simulink model "RABBIT_sfunction_test"  (R2015a)
settings: Solver=FixedStepDiscrete  StartTime=t_start  StopTime=t_end  FixedStep=dt  RelTol=1e-3
undefined symbols (not defined in the file or in its folder): dt
libraries: RABBIT_lib x2
settings Model: Creator=ffelici  LastModifiedBy=ffelici
settings OptimizationCC: OptimizeModelRefInitCode=on  LifeSpan=1
settings HardwareCC: TargetBitPerLong=64  TargetBitPerPointer=64  TargetLongLongMode=on  TargetIntDivRoundTo=Zero  TargetEndianess=LittleEndian  TargetWordSize=64  TargetHWDeviceType=MATLAB Host  ProdEqTarget=off
settings RTWCC: SystemTargetFile=ert_shrlib.tlc  TemplateMakefile=ert_unix_rabbit.tmf  Description=Embedded Coder (host-based shared library target)  RetainRTWFile=on  BuildConfiguration=Specify  RTWCompilerOptimization=Custom
settings CodeAppCC: IgnoreCustomStorageClasses=off
settings STFCustomTargetCC: GenerateSampleERTMain=off  ParMdlRefBuildCompliant=on  CompOptLevelCompliant=on  CombineOutputUpdateFcns=on  SupportContinuousTime=off  SupportNonInlinedSFcns=on  SupportVariableSizeSignals=off  ModelStepFunctionPrototypeControlCompliant=on  SystemTargetFile=ert_shrlib.tlc
settings ERTTargetCC: GenerateSampleERTMain=off  ParMdlRefBuildCompliant=on  CompOptLevelCompliant=on  SupportContinuousTime=off  SupportNonInlinedSFcns=on  SupportVariableSizeSignals=off  ModelStepFunctionPrototypeControlCompliant=on  ERTCustomFileTemplate=example_file_process.tlc

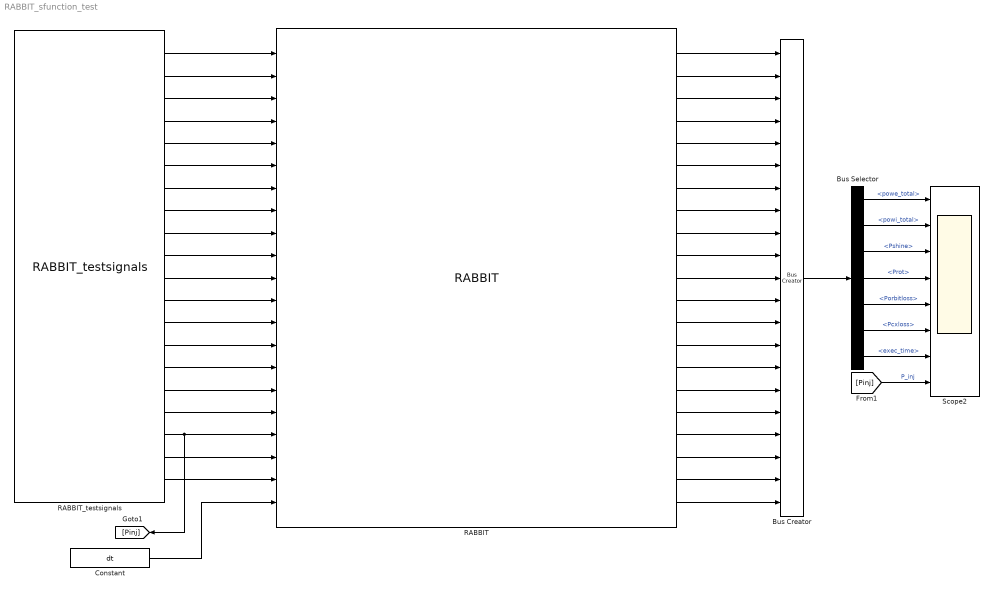
== system RABBIT_sfunction_test ==
  Bus Creator : BusCreator  Inputs=21
  Bus Selector : BusSelector  OutputSignals=powe_total,powi_total,Pshine,Prot,Porbitloss,Pcxloss,exec_time
  Constant : Constant  Value=dt
  RABBIT : RABBIT_lib/RABBIT  RABBITparams=RABBITparams
  RABBIT_testsignals : RABBIT_lib/RABBIT_testsignals  RABBITsignals=RABBITsignals  dt=dt
  Scope2 : Scope  NumInputPorts=8
      settings: YMin=0~0~600000~350000~-1~-1.25e-10~-1~-5  YMax=100000~250000~950000~550000~1~5e-11~1~5
  wires:
  Bus Selector/1 -> Scope2/1  "<powe_total>"
  Bus Selector/2 -> Scope2/2  "<powi_total>"
  Bus Selector/3 -> Scope2/3  "<Pshine>"
  Bus Selector/4 -> Scope2/4  "<Prot>"
  Bus Selector/5 -> Scope2/5  "<Porbitloss>"
  Bus Selector/6 -> Scope2/6  "<Pcxloss>"
  Bus Selector/7 -> Scope2/7  "<exec_time>"
  [Pinj] -> Scope2/8  "P_inj"
  Bus Creator/1 -> Bus Selector/1
  Constant/1 -> RABBIT/21
  RABBIT_testsignals/20 -> RABBIT/20
  RABBIT_testsignals/19 -> RABBIT/19
  RABBIT_testsignals/17 -> RABBIT/17
  RABBIT_testsignals/18 -> RABBIT/18, [Pinj]
  RABBIT_testsignals/16 -> RABBIT/16
  RABBIT_testsignals/15 -> RABBIT/15
  RABBIT_testsignals/14 -> RABBIT/14
  RABBIT_testsignals/13 -> RABBIT/13
  RABBIT_testsignals/12 -> RABBIT/12
  RABBIT_testsignals/11 -> RABBIT/11
  RABBIT_testsignals/10 -> RABBIT/10
  RABBIT_testsignals/9 -> RABBIT/9
  RABBIT_testsignals/8 -> RABBIT/8
  RABBIT_testsignals/7 -> RABBIT/7
  RABBIT_testsignals/6 -> RABBIT/6
  RABBIT_testsignals/4 -> RABBIT/4
  RABBIT_testsignals/5 -> RABBIT/5
  RABBIT_testsignals/3 -> RABBIT/3
  RABBIT_testsignals/2 -> RABBIT/2
  RABBIT_testsignals/1 -> RABBIT/1
  RABBIT/1 -> Bus Creator/1
  RABBIT/2 -> Bus Creator/2
  RABBIT/3 -> Bus Creator/3
  RABBIT/4 -> Bus Creator/4
  RABBIT/21 -> Bus Creator/21
  RABBIT/20 -> Bus Creator/20
  RABBIT/19 -> Bus Creator/19
  RABBIT/18 -> Bus Creator/18
  RABBIT/17 -> Bus Creator/17
  RABBIT/16 -> Bus Creator/16
  RABBIT/15 -> Bus Creator/15
  RABBIT/14 -> Bus Creator/14
  RABBIT/13 -> Bus Creator/13
  RABBIT/12 -> Bus Creator/12
  RABBIT/11 -> Bus Creator/11
  RABBIT/10 -> Bus Creator/10
  RABBIT/9 -> Bus Creator/9
  RABBIT/8 -> Bus Creator/8
  RABBIT/7 -> Bus Creator/7
  RABBIT/5 -> Bus Creator/5
  RABBIT/6 -> Bus Creator/6
